simulink model "external_mode_serial_am13x"  (R2025b)
settings: Solver=FixedStepAuto  StartTime=0.0  StopTime=20  RelTol=1e-3  EnableMultiTasking=on
libraries: simulink x3
settings Model: SimulationMode=processor-in-the-loop (pil)  CodeVerificationMode=processor-in-the-loop (pil)  Creator=a1255762  LastModifiedBy=a1255762
settings OptimizationCC: DefaultUnderspecifiedDataType=single  EnhancedBackFolding=on  PassReuseOutputArgsAs=Individual arguments  ZeroExternalMemoryAtStartup=off  ZeroInternalMemoryAtStartup=off  MaxStackSize=64  OptimizeBlockOrder=speed  DifferentSizesBufferReuse=on  OptimizationCustomize=off  EfficientTunableParamExpr=on
settings DebuggingCC: ParameterPrecisionLossMsg=none  ParameterTunabilityLossMsg=error
settings HardwareCC: ProdBitPerPointer=32.0  ProdBitPerSizeT=32.0  ProdBitPerPtrDiffT=32.0  ProdLargestAtomicInteger=Long  ProdLargestAtomicFloat=Double  ProdWordSize=32.0  ProdLongLongMode=on  ProdHWDeviceType=ARM Compatible->ARM Cortex
settings SFSimCC: MATLABDynamicMemAlloc=off
settings RTWCC: SystemTargetFile=ert.tlc  HardwareBoard=AM13E230x  TemplateMakefile=ert_default_tmf  GenerateReport=on  Toolchain=TI ARM Clang Compiler AM13x | gmake  BuildConfiguration=Debug  IncludeHyperlinkInReport=on  LaunchReport=on  CodeExecutionProfiling=on  GenerateTraceInfo=on  GenerateCodeReplacementReport=on  Description=Embedded Coder
settings CodeAppCC: ForceParamTrailComments=on  IgnoreCustomStorageClasses=off  MaxIdLength=256.0  OperatorAnnotations=on  SimulinkDataObjDesc=on  SFDataObjDesc=on  InsertBlockDesc=on
settings ERTTargetCC: ExtModeTransport=3.0  ExtModeStaticAlloc=on  ExtModeMexFile=ext_xcp  ExtModeIntrfLevel=Level2 - Open  InlinedParameterPlacement=Hierarchical  ERTCustomFileTemplate=AM13x_codertarget_file_process.tlc  CodeReplacementLibrary=AM13x_TMU

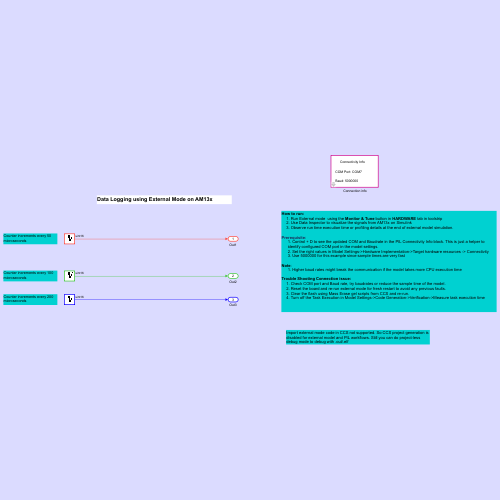
[thumbnail: Simulink's stored preview of the top-level diagram]
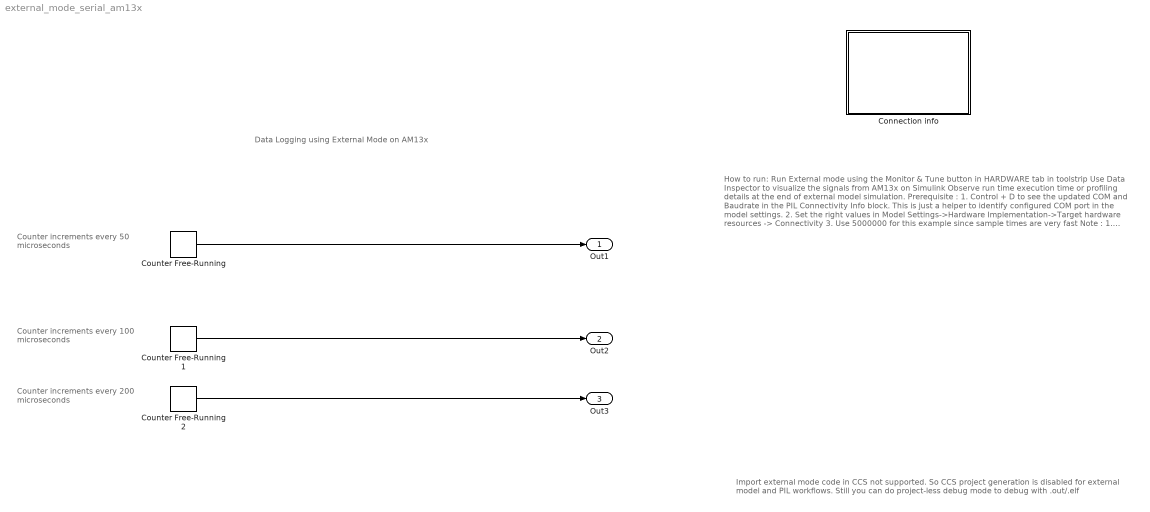
== system external_mode_serial_am13x ==
  note: How to run:
      | Run External mode using the Monitor & Tune button in HARDWARE tab in toolstrip
      | Use Data Inspector to visualize the signals from AM13x on Simulink
      | Observe run time execution time or profiling details at the end of external model simulation.
      |
      | Prerequisite :
      | 1. Control + D to see the updated COM and Baudrate in the PIL Connectivity Info block. This is just a helper to identify configured COM port in the model settings.
      | 2. Set the right values in Model Settings->Hardware Implementation->Target hardware resources -> Connectivity
      | 3. Use 5000000 for this example since sample times are very fast
      |
      | Note :
      | 1. Higher baud rates might break the communication if the model takes more CPU execution time
      |
      | Trouble Shooting Connection issue:
      | Check COM port and Baud rate, try baudrates or reduce the sample time of the model.
      | Reset the board and re-run external mode for fresh restart to avoid any previous faults.
      | Clear the flash using Mass Erase gel scripts from CCS and re-run.
      | Turn off the Task Execution in Model Settings->Code Generation->Verification->Measure task execution time
  note: Data Logging using External Mode on AM13x
  note: Counter increments every 50 microseconds
  note: Counter increments every 100 microseconds
  note: Counter increments every 200 microseconds
  note: Import external mode code in CCS not supported. So CCS project generation is disabled for external model and PIL workflows. Still you can do project-less debug mode to debug with .out/.elf
  " Connection info" : Subsystem  mask{Parameter1=|}
      mask Parameter1=|
      | codertarget.data.setParameterValue(bdroot, 'Connection.Serialport', 'COM3')
      | codertarget.data.setParameterValue(bdroot, 'Connection.Baud', '5000000')
      mask prompts: Parameter1 "Change programmatically"
      mask Display:
      | % Update mask parameters with current values when opened
      | 
      | pilData = codertarget.data.getParameterValue(bdroot, 'Connection');
      | 
      | 
      | % Use text() function with specific positioning
      | text(0.2, 0.8, 'Connectivity Info', 'HorizontalAlignment', 'left');
      | text(0.1, 0.5, ['COM Port: ' pilData.Serialport], 'HorizontalAlignment', 'left');
      | text(0.1, 0.2, ['Baud: ' pilData.Baud], 'HorizontalAlignment', 'left');
  Counter Free-Running : simulink/Sources/Counter Free-Running  NumBits=16  tsamp=50e-6
  Counter Free-Running1 : simulink/Sources/Counter Free-Running  NumBits=16  tsamp=100e-6
  Counter Free-Running2 : simulink/Sources/Counter Free-Running  NumBits=16  tsamp=200e-6
  Out1 : Outport
  Out2 : Outport  Port=2
  Out3 : Outport  Port=3
  wires:
  Counter Free-Running/1 -> Out1/1
  Counter Free-Running1/1 -> Out2/1
  Counter Free-Running2/1 -> Out3/1

== system external_mode_serial_am13x/ Connection info ==
